simulink model "Cuadcoptero_12estados"  (R2015a)
settings: Solver=ode45  StartTime=0.0  StopTime=50  RelTol=1e-3
values from neighbouring files (symbols this model uses):
  b = 2.64e-4    (= 0.000264)    [ParametrosQuadcoptero.m]
  d = 7.5e-7    (= 7.5e-07)    [ParametrosQuadcoptero.m]
  g = 9.81    [ParametrosQuadcoptero.m]
  Ix = 0.033    [ParametrosQuadcoptero.m]
  Iy = 0.033    [ParametrosQuadcoptero.m]
  Iz = 0.066    [ParametrosQuadcoptero.m]
  L = 0.5    [ParametrosQuadcoptero.m]
  m = 4    [ParametrosQuadcoptero.m]
  Ts = 0.05    [ModeloVariablesEstado.m]
  x10_0 = 0    [CondicionesIniciales.m]
  x11_0 = 0    [CondicionesIniciales.m]
  x12_0 = 0    [CondicionesIniciales.m]
  x1_0 = 0    [CondicionesIniciales.m]
  x2_0 = 0    [CondicionesIniciales.m]
  x3_0 = 0    [CondicionesIniciales.m]
  x4_0 = 0    [CondicionesIniciales.m]
  x5_0 = 10    [CondicionesIniciales.m]
  x6_0 = 0    [CondicionesIniciales.m]
  x7_0 = 0    [CondicionesIniciales.m]
  x8_0 = 0    [CondicionesIniciales.m]
  x9_0 = 0    [CondicionesIniciales.m]
libraries: mpclib x1
settings Model: Creator=Dell  LastModifiedBy=Dell

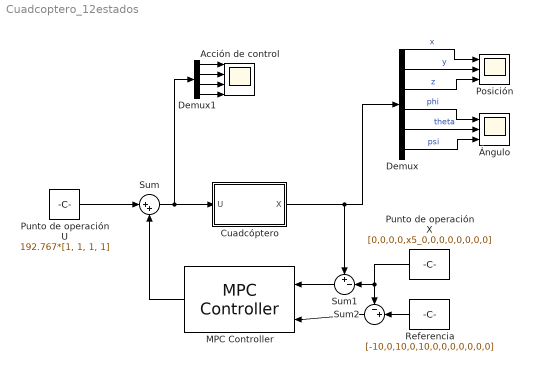
== system Cuadcoptero_12estados ==
  Acción de control : Scope  NumInputPorts=4
      settings: YMin=-5~-5~-5~-5  YMax=5~5~5~5  SaveName=ScopeData2
  Cuadcóptero : Subsystem
  Demux : Demux  Outputs=12
  Demux1 : Demux
  MPC Controller : mpclib/MPC Controller  SCDEnableBlockLinearizationSpecification=on  mpcobj=MPC1  is_multiple=0  enable_value=0  n_mv=4  n_mo=12  n_md=0  n_ts=0.05  is_designfromscratch=0  return_u0=off  ref_from_ws=off  ref_signal_name=[]  ref_preview=off  md_from_ws=off  md_signal_name=[]  md_preview=off  from_project=off  project_file=MPCtask.mat  md_inport=off  mv_inport=off  cost_outport=off  return_sequence=off  return_qpstatus=off  return_state=off  state_inport=off  lims_inport=off  ywt_inport=off  uwt_inport=off  duwt_inport=off  rhoeps_inport=off  uref_inport=off  BlockDataType=double  SampleTimeInherited=off  switch_inport=off
  Posición : Scope  NumInputPorts=3
      settings: YMin=-5~-5~-5  YMax=5~5~5
  Punto de operación U : Constant  Value=192.767*[1, 1, 1, 1]
  Punto de operación X : Constant  Value=[0,0,0,0,x5_0,0,0,0,0,0,0,0]  SampleTime=Ts
  Referencia : Constant  Value=[-10,0,10,0,10,0,0,0,0,0,0,0]  SampleTime=Ts
  Sum : Sum  Inputs=|++
  Sum1 : Sum  Inputs=+-|
  Sum2 : Sum  Inputs=-+|
  Ángulo : Scope  NumInputPorts=3
      settings: YMin=-5~-5~-5  YMax=5~5~5
  wires:
  Demux/1 -> Posición/1  "x"
  Demux/3 -> Posición/2  "y"
  Demux/5 -> Posición/3  "z"
  Demux/7 -> Ángulo/1  "phi"
  Demux/9 -> Ángulo/2  "theta"
  Demux/11 -> Ángulo/3  "psi"
  Cuadcóptero/1(X) -> Demux/1, Sum1/1
  Punto de operación U/1 -> Sum/1
  Sum/1 -> Demux1/1, Cuadcóptero/1(U)
  MPC Controller/1 -> Sum/2
  Sum1/1 -> MPC Controller/1
  Punto de operación X/1 -> Sum2/1, Sum1/2
  Referencia/1 -> Sum2/2
  Sum2/1 -> MPC Controller/2
  Demux1/1 -> Acción de control/1
  Demux1/2 -> Acción de control/2
  Demux1/3 -> Acción de control/3
  Demux1/4 -> Acción de control/4

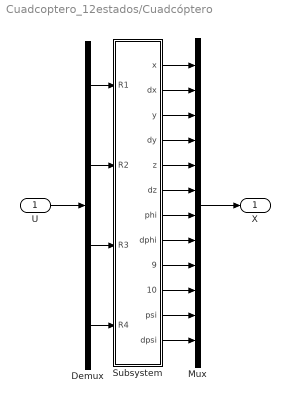
== system Cuadcoptero_12estados/Cuadcóptero ==
  U : Inport
  Demux : Demux
  Mux : Mux  Inputs=12
  Subsystem : Subsystem
  X : Outport
  wires:
  Subsystem/4(dy) -> Mux/4
  Subsystem/5(z) -> Mux/5
  U/1 -> Demux/1
  Subsystem/7(phi) -> Mux/7
  Subsystem/10(dtheta) -> Mux/10
  Subsystem/12(dpsi) -> Mux/12
  Subsystem/9(theta) -> Mux/9
  Subsystem/8(dphi) -> Mux/8
  Subsystem/6(dz) -> Mux/6
  Subsystem/11(psi) -> Mux/11
  Demux/4 -> Subsystem/4(R4)
  Subsystem/3(y) -> Mux/3
  Demux/2 -> Subsystem/2(R2)
  Demux/3 -> Subsystem/3(R3)
  Subsystem/1(x) -> Mux/1
  Subsystem/2(dx) -> Mux/2
  Mux/1 -> X/1
  Demux/1 -> Subsystem/1(R1)

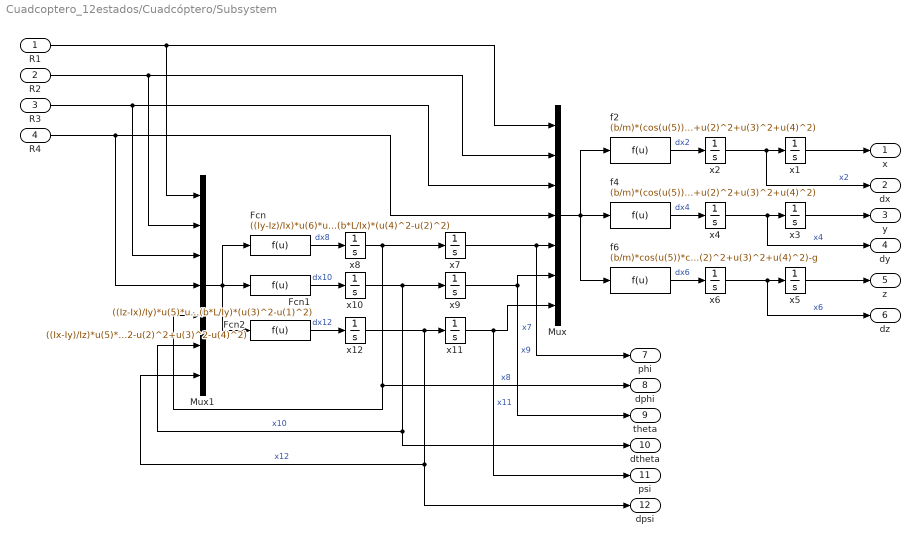
== system Cuadcoptero_12estados/Cuadcóptero/Subsystem ==
  R1 : Inport
  R2 : Inport  Port=2
  R3 : Inport  Port=3
  R4 : Inport  Port=4
  Fcn : Fcn  Expr=((Iy-Iz)/Ix)*u(6)*u(7)+(b*L/Ix)*(u(4)^2-u(2)^2)
  Fcn1 : Fcn  Expr=((Iz-Ix)/Iy)*u(5)*u(7)+(b*L/Iy)*(u(3)^2-u(1)^2)
  Fcn2 : Fcn  Expr=((Ix-Iy)/Iz)*u(5)*u(6)+(d/Iz)*(u(1)^2-u(2)^2+u(3)^2-u(4)^2)
  Mux : Mux  Inputs=7
  Mux1 : Mux  Inputs=7
  f2 : Fcn  Expr=(b/m)*(cos(u(5))*sin(u(6))*cos(u(7))+sin(u(5))*sin(u(7)))*(u(1)^2+u(2)^2+u(3)^2+u(4)^2)
  f4 : Fcn  Expr=(b/m)*(cos(u(5))*sin(u(6))*sin(u(7))-sin(u(5))*cos(u(7)))*(u(1)^2+u(2)^2+u(3)^2+u(4)^2)
  f6 : Fcn  Expr=(b/m)*cos(u(5))*cos(u(6))*(u(1)^2+u(2)^2+u(3)^2+u(4)^2)-g
  x1 : Integrator  InitialCondition=x1_0
  x10 : Integrator  InitialCondition=x10_0
  x11 : Integrator  InitialCondition=x11_0
  x12 : Integrator  InitialCondition=x12_0
  x2 : Integrator  InitialCondition=x2_0
  x3 : Integrator  InitialCondition=x3_0
  x4 : Integrator  InitialCondition=x4_0
  x5 : Integrator  InitialCondition=x5_0
  x6 : Integrator  InitialCondition=x6_0
  x7 : Integrator  InitialCondition=x7_0
  x8 : Integrator  InitialCondition=x8_0
  x9 : Integrator  InitialCondition=x9_0
  x : Outport
  dx : Outport  Port=2
  y : Outport  Port=3
  dy : Outport  Port=4
  z : Outport  Port=5
  dz : Outport  Port=6
  phi : Outport  Port=7
  dphi : Outport  Port=8
  theta : Outport  Port=9
  dtheta : Outport  Port=10
  psi : Outport  Port=11
  dpsi : Outport  Port=12
  wires:
  Fcn2/1 -> x12/1  "dx12"
  f6/1 -> x6/1  "dx6"
  Mux/1 -> f6/1, f2/1, f4/1
  R4/1 -> Mux1/4, Mux/4
  R1/1 -> Mux1/1, Mux/1
  f4/1 -> x4/1  "dx4"
  x12/1 -> x11/1, dpsi/1, Mux1/7  "x12"
  x1/1 -> x/1
  R2/1 -> Mux1/2, Mux/2
  Fcn/1 -> x8/1  "dx8"
  f2/1 -> x2/1  "dx2"
  x2/1 -> dx/1, x1/1  "x2"
  x8/1 -> dphi/1, Mux1/5, x7/1  "x8"
  x11/1 -> psi/1, Mux/7  "x11"
  Mux1/1 -> Fcn1/1, Fcn/1, Fcn2/1
  x3/1 -> y/1
  Fcn1/1 -> x10/1  "dx10"
  x10/1 -> x9/1, dtheta/1, Mux1/6  "x10"
  x7/1 -> phi/1, Mux/5  "x7"
  x5/1 -> z/1
  x4/1 -> dy/1, x3/1  "x4"
  x6/1 -> dz/1, x5/1  "x6"
  x9/1 -> theta/1, Mux/6  "x9"
  R3/1 -> Mux1/3, Mux/3
